simulink model "LSLRecieverSimulink"  (R2023a)
settings: Solver=FixedStepAuto  StartTime=0.0  StopTime=inf  FixedStep=1/250  RelTol=1e-3
libraries: FeatureExtraction x1, simulink x1, LSL x1, Tools x1, Transformation x1, Visualization x1
settings Model: Creator=sieghartsleitner  LastModifiedBy=wong

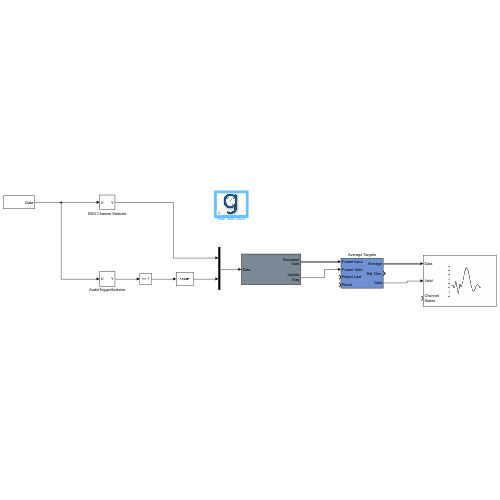
[thumbnail: Simulink's stored preview of the top-level diagram]
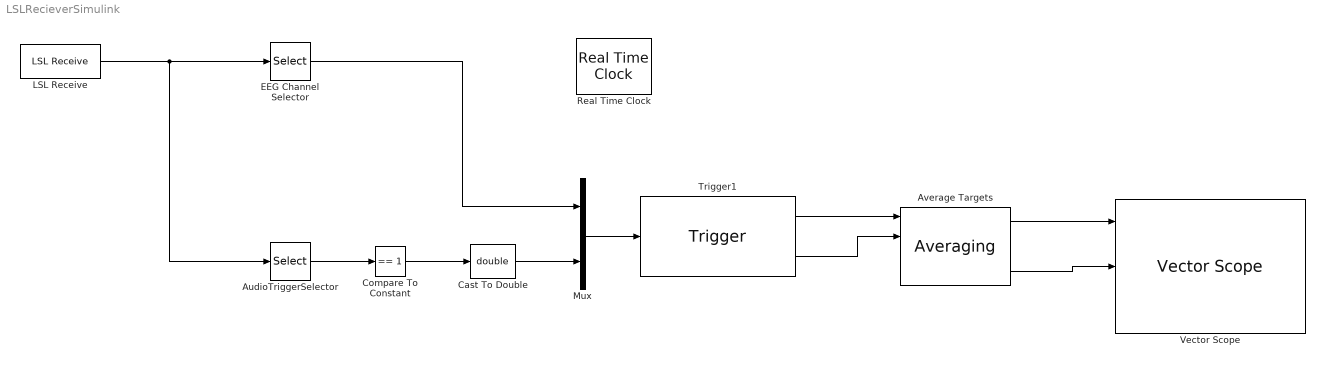
== system LSLRecieverSimulink ==
  AudioTriggerSelector : Selector  InputPortWidth=10  IndexOptions=Index vector (dialog)  Indices=[9]  OutputSizes=1
  Average Targets : FeatureExtraction/Averaging  mode_select=1 - average all data  mode=0  window=3  add_std=on  do_baseline_correction=off  baseline_interval=[-0 0]  sampletime=1/250
      settings: SourceProductName=g.HIsys
  Cast To Double : DataTypeConversion  OutDataTypeStr=double  SaturateOnIntegerOverflow=off  RndMeth=Floor
  Compare To Constant : simulink/Logic and Bit Operations/Compare To Constant  relop===  const=1  OutDataTypeStr=boolean
  EEG Channel Selector : Selector  InputPortWidth=10  IndexOptions=Index vector (dialog)  Indices=[1]  OutputSizes=1
  LSL Receive : LSL/LSL Receive  noChannels=10  lslPropName=name  lslPropValue='EEG'  sampleRate=250  signalSource=off
      settings: SourceProductName=g.HIsys
  Mux : Mux  Inputs=2
  Real Time Clock : Tools/Real Time Clock  timeprofile=off
      settings: SourceProductName=g.HIsys
  Trigger1 : Transformation/Trigger  trigchan=2  edge_select=RISING  edge=0  treshold=1  ext_treshold=off  windowsize=0.9  pretrigger=-0.2  sampletime=1/250  validity_select=STANDARD (global validity flag for all channels)  validity=0  discardTriggerChannels=on
      settings: SourceProductName=g.HIsys
  Vector Scope : Visualization/Vector Scope
      settings: SourceProductName=g.HIsys
  wires:
  LSL Receive/1 -> EEG Channel Selector/1, AudioTriggerSelector/1
  AudioTriggerSelector/1 -> Compare To Constant/1
  EEG Channel Selector/1 -> Mux/1
  Compare To Constant/1 -> Cast To Double/1
  Cast To Double/1 -> Mux/2
  Trigger1/1 -> Average Targets/1
  Trigger1/2 -> Average Targets/2
  Average Targets/1 -> Vector Scope/1
  Mux/1 -> Trigger1/1
  Average Targets/3 -> Vector Scope/2
